simulink model "Tarea1Parte1SeccionEii"  (R2021a)
settings: Solver=VariableStepAuto  StartTime=0.0  StopTime=10.0  RelTol=1e-3
values from neighbouring files (symbols this model uses):
  Kd = -139.132    [Tarea1Parte1SeccionE.m]
  Kvs = 0.001    [Tarea1_Parte1_Todaslassecciones.m]    (also in Tarea1parte1SeccionD.m; simulink.m)
  T = 215.664    [Tarea1Parte1SeccionE.m]    (also in Tarea1_Parte1_Todaslassecciones.m)
undefined symbols (not defined in the file or in its folder): K
settings Model: Creator=Royer  LastModifiedBy=Royer

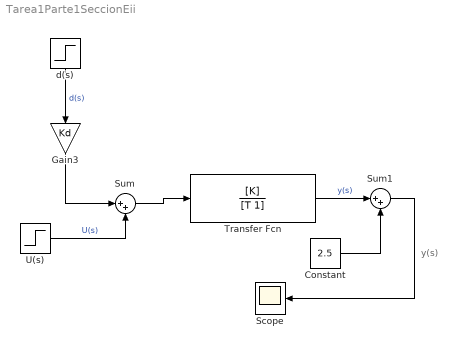
== system Tarea1Parte1SeccionEii ==
  note: y(s)
  Constant : Constant  Value=2.5
  Gain3 : Gain  Gain=Kd
  Scope : Scope
  Sum : Sum  Inputs=|++
  Sum1 : Sum  Inputs=|++
  Transfer Fcn : TransferFcn  Numerator=[K]  Denominator=[T 1]
  U(s) : Step  Before=100  SampleTime=0
  d(s) : Step  Before=Kvs  SampleTime=0
  wires:
  Gain3/1 -> Sum/1
  d(s)/1 -> Gain3/1  "d(s)"
  Sum/1 -> Transfer Fcn/1
  U(s)/1 -> Sum/2  "U(s)"
  Transfer Fcn/1 -> Sum1/1  "y(s)"
  Constant/1 -> Sum1/2
  Sum1/1 -> Scope/1
